simulink model "motor_pid"  (R2018b)
settings: Solver=FixedStepAuto  StartTime=0.0  StopTime=10.0  RelTol=1e-3
values from neighbouring files (symbols this model uses):
  Kd = 0    [motorspace.mat]    (also in pid_init.m = -1.83138864157e-05)
  Ki = 0.109445430355    [motorspace.mat]    (also in pid_init.m = 3.51141025885)
  Kp = 0.00296411720747    [motorspace.mat]    (also in pid_init.m = 0.0314554077959)
  OutputLimitMax = inf    [motorspace.mat]
  OutputLimitMin = 0    [motorspace.mat]
settings Model: Creator=tengo  LastModifiedBy=tengo

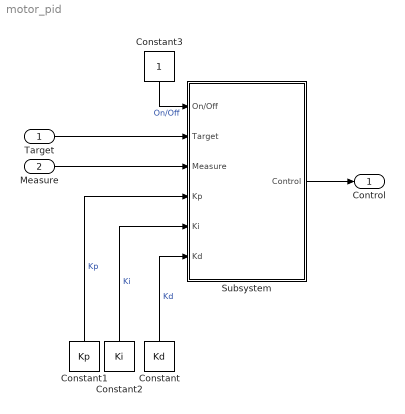
== system motor_pid ==
  Target : Inport
  Measure : Inport  Port=2
  Constant : Constant  Value=Kd
  Constant1 : Constant  Value=Kp
  Constant2 : Constant  Value=Ki
  Constant3 : Constant
  Subsystem : Subsystem
  Control : Outport
  wires:
  Target/1 -> Subsystem/2(Target)
  Measure/1 -> Subsystem/3(Measure)
  Subsystem/1(Control) -> Control/1
  Constant/1 -> Subsystem/6(Kd)  "Kd"
  Constant2/1 -> Subsystem/5(Ki)  "Ki"
  Constant1/1 -> Subsystem/4(Kp)  "Kp"
  Constant3/1 -> Subsystem/1(On/Off)  "On/Off"

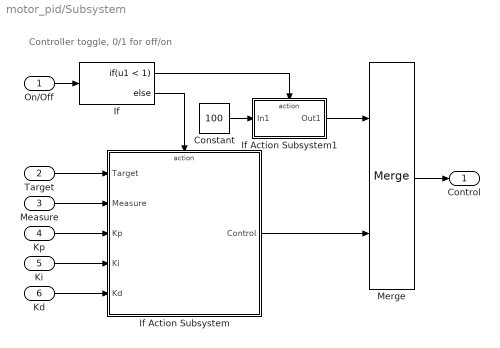
== system motor_pid/Subsystem ==
  note: Controller toggle, 0/1 for off/on
  On/Off : Inport
  Target : Inport  Port=2
  Measure : Inport  Port=3
  Kp : Inport  Port=4
  Ki : Inport  Port=5
  Kd : Inport  Port=6
  Constant : Constant  Value=100
  If : If  IfExpression=u1 < 1
  If Action Subsystem : Subsystem  TreatAsAtomicUnit=on
  If Action Subsystem1 : Subsystem  TreatAsAtomicUnit=on
  Merge : Merge
  Control : Outport
  wires:
  If/2 -> If Action Subsystem/Action
  If Action Subsystem/1(Control) -> Merge/2
  Merge/1 -> Control/1
  On/Off/1 -> If/1
  If/1 -> If Action Subsystem1/Action
  Constant/1 -> If Action Subsystem1/1(In1)
  If Action Subsystem1/1(Out1) -> Merge/1
  Kp/1 -> If Action Subsystem/3(Kp)
  Ki/1 -> If Action Subsystem/4(Ki)
  Kd/1 -> If Action Subsystem/5(Kd)
  Measure/1 -> If Action Subsystem/2(Measure)
  Target/1 -> If Action Subsystem/1(Target)

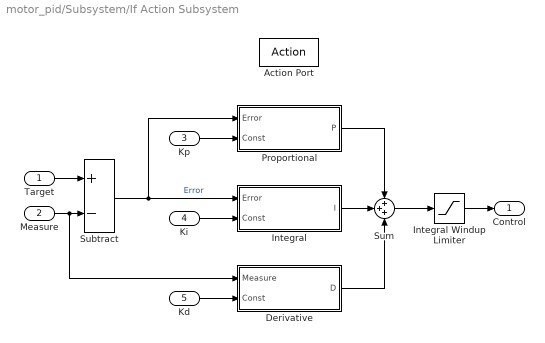
== system motor_pid/Subsystem/If Action Subsystem ==
  Target : Inport
  Measure : Inport  Port=2
  Kp : Inport  Port=3
  Ki : Inport  Port=4
  Kd : Inport  Port=5
  Action Port : ActionPort  ActionType=else
  Derivative : Subsystem
  Integral : Subsystem
  Integral Windup Limiter : Saturate  UpperLimit=OutputLimitMax  LowerLimit=OutputLimitMin
  Proportional : Subsystem
  Subtract : Sum  Inputs=+-
  Sum : Sum  Inputs=3
  Control : Outport
  wires:
  Measure/1 -> Derivative/1(Measure), Subtract/2
  Ki/1 -> Integral/2(Const)
  Target/1 -> Subtract/1
  Proportional/1(P) -> Sum/1
  Kp/1 -> Proportional/2(Const)
  Derivative/1(D) -> Sum/3
  Integral/1(I) -> Sum/2
  Kd/1 -> Derivative/2(Const)
  Subtract/1 -> Proportional/1(Error), Integral/1(Error)  "Error"
  Sum/1 -> Integral Windup Limiter/1
  Integral Windup Limiter/1 -> Control/1

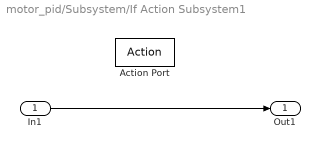
== system motor_pid/Subsystem/If Action Subsystem1 ==
  In1 : Inport
  Action Port : ActionPort  ActionType=then
  Out1 : Outport
  wires:
  In1/1 -> Out1/1

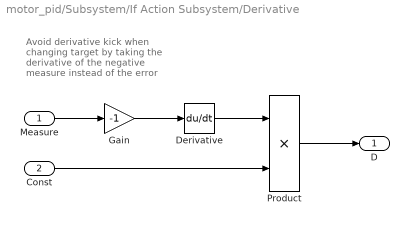
== system motor_pid/Subsystem/If Action Subsystem/Derivative ==
  note: Avoid derivative kick when
      | changing target by taking the
      | derivative of the negative
      | measure instead of the error
  Measure : Inport
  Const : Inport  Port=2
  Derivative : Derivative
  Gain : Gain  Gain=-1
  Product : Product
  D : Outport
  wires:
  Measure/1 -> Gain/1
  Const/1 -> Product/2
  Product/1 -> D/1
  Derivative/1 -> Product/1
  Gain/1 -> Derivative/1

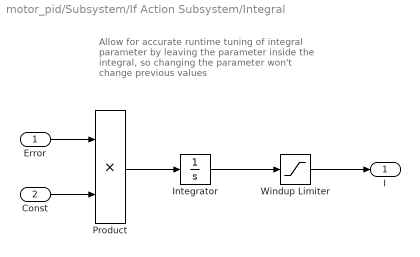
== system motor_pid/Subsystem/If Action Subsystem/Integral ==
  note: Allow for accurate runtime tuning of integral
      | parameter by leaving the parameter inside
      | the integral, so changing the parameter won't
      | change previous values
  Error : Inport
  Const : Inport  Port=2
  Integrator : Integrator
  Product : Product
  Windup Limiter : Saturate  UpperLimit=OutputLimitMax  LowerLimit=OutputLimitMin
  I : Outport
  wires:
  Product/1 -> Integrator/1
  Error/1 -> Product/1
  Const/1 -> Product/2
  Integrator/1 -> Windup Limiter/1
  Windup Limiter/1 -> I/1

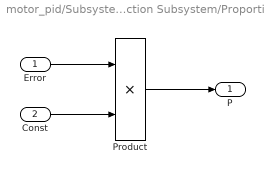
== system motor_pid/Subsystem/If Action Subsystem/Proportional ==
  Error : Inport
  Const : Inport  Port=2
  Product : Product
  P : Outport
  wires:
  Const/1 -> Product/2
  Error/1 -> Product/1
  Product/1 -> P/1
